simulink model "PID_SingleTank"  (R2016b)
settings: Solver=ode5  StartTime=0.0  StopTime=600  FixedStep=0.1  MaxStep=0.1  RelTol=1e-3
PreLoadFcn:
  | FuzzyK=readfis('FuzzySugenoPID_SingleTank.fis');
StartFcn:
  | FuzzyK=readfis('FuzzySugenoPID_SingleTank.fis');
Description:
  | The model describes dynamic properties of tank level system. The differential equation is:
  |                                            d/dt{Ah(t))=ku(t)-a*sqrt(2*g*h(t))
settings Model: ExtModeTrigMode=oneshot  ExtModeArmWhenConnect=off  Creator=Huynh Thai Hoang  LastModifiedBy=HTH
settings SolverCC: InitialStep=0.1
settings DataIOCC: SaveFormat=Array  SignalLoggingSaveFormat=ModelDataLogs  SaveOutput=off  SaveTime=off  SignalLoggingName=sigsOut
settings OptimizationCC: BooleanDataType=off  ExpressionDepthLimit=2147483647  LifeSpan=inf
settings DebuggingCC: SaveWithParameterizedLinksMsg=none  UnderspecifiedInitializationDetection=Classic  MergeDetectMultiDrivingBlocksExec=none  SignalResolutionControl=TryResolveAllWithWarning  MultiTaskDSMMsg=warning  MultiTaskCondExecSysMsg=none  FcnCallInpInsideContextMsg=warning  StateNameClashWarn=warning  SFUnexpectedBacktrackingDiag=warning  SFNoUnconditionalDefaultTransitionDiag=warning  SFExecutionAtInitializationDiag=none
settings HardwareCC: ProdBitPerPointer=32  ProdBitPerSizeT=32  ProdBitPerPtrDiffT=32  ProdLargestAtomicFloat=None  ProdIntDivRoundTo=Undefined  ProdEndianess=Unspecified  ProdWordSize=32  ProdHWDeviceType=32-bit Generic  TargetUnknown=on
settings ModelReferenceCC: PropagateSignalLabelsOutOfModel=off
settings GRTTargetCC: TargetLangStandard=C89/C90 (ANSI)  GeneratePreprocessorConditionals=Disable all  CombineOutputUpdateFcns=off  GRTInterface=on
settings ConfigComp: CovMetricSettings=dw  CovHtmlReporting=on  CovSaveCumulativeToWorkspaceVar=on  CovSaveSingleToWorkspaceVar=on  CovExternalEMLEnable=off

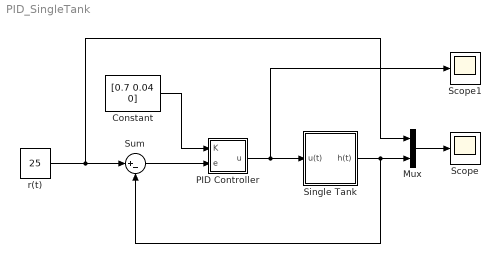
== system PID_SingleTank ==
  Constant : Constant  Value=[0.7 0.04 0]
  Mux : Mux  Inputs=2
  PID Controller : Subsystem  AncestorBlock=simulink_extras/Additional Linear/PID Controller  mask(PID Controller){}
      mask help:
      | Enter expressions for proportional, integral, and derivative terms.
      | P+I/s+Ds
      mask Help: This block implements a PID controller where parameters are entered for the Proportional, Integral and Derivative terms. Unmask this block to see how it works. The derivative term is implemented using a true derivative block.
  Scope : Scope
  Scope1 : Scope
  Single Tank : Subsystem  mask{A_min=50, A_max=200, a_out=1, h_max=50, Q_max=300, U_max=12, C=0.6}
      mask prompts: A_min "Minimum cross area (cm2)"; A_max "Maximum cross area (cm2)"; a_out "Outlet area (cm2)"; h_max "Tank height (cm)"; Q_max "Maximum pump flow (cm3/sec)"; U_max "Maximum control voltage (V)"; C "Discharge constant"
      mask init:
      | g=981;
      | k=Q_max/U_max;
      mask Display:
      | plot([0.1 0.3 0.9],[0.9 0.1 0.1]);
      | plot([0.9 0.7 0.9],[0.9 0.2 0.2]);
  Sum : Sum  Inputs=|+-  SaturateOnIntegerOverflow=on
  r(t) : Constant  Value=25
  wires:
  r(t)/1 -> Sum/1, Mux/1
  Sum/1 -> PID Controller/2(e)
  PID Controller/1(u) -> Single Tank/1(u(t)), Scope1/1
  Single Tank/1(h(t)) -> Sum/2, Mux/2
  Constant/1 -> PID Controller/1(K)
  Mux/1 -> Scope/1

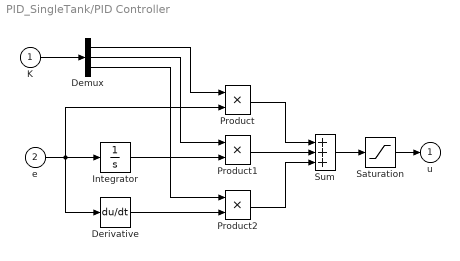
== system PID_SingleTank/PID Controller ==
  K : Inport
  e : Inport  Port=2
  Demux : Demux  Outputs=3
  Derivative : Derivative
  Integrator : Integrator
  Product : Product  SaturateOnIntegerOverflow=on  OutDataTypeStr=Inherit: Same as first input
  Product1 : Product  SaturateOnIntegerOverflow=on  OutDataTypeStr=Inherit: Same as first input
  Product2 : Product  SaturateOnIntegerOverflow=on  OutDataTypeStr=Inherit: Same as first input
  Saturation : Saturate  UpperLimit=12  LowerLimit=0
  Sum : Sum  Inputs=+++  SaturateOnIntegerOverflow=on  InputSameDT=on  OutDataTypeStr=Inherit: Same as first input
  u : Outport  InitialOutput=0
  wires:
  Product/1 -> Sum/1
  e/1 -> Product/2, Integrator/1, Derivative/1
  Sum/1 -> Saturation/1
  K/1 -> Demux/1
  Demux/1 -> Product/1
  Product1/1 -> Sum/2
  Integrator/1 -> Product1/2
  Demux/2 -> Product1/1
  Derivative/1 -> Product2/2
  Product2/1 -> Sum/3
  Demux/3 -> Product2/1
  Saturation/1 -> u/1

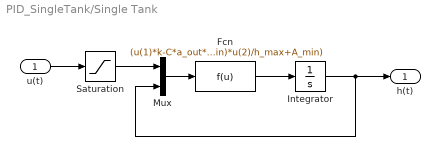
== system PID_SingleTank/Single Tank ==
  u(t) : Inport
  Fcn : Fcn  Expr=(u(1)*k-C*a_out*sqrt(2*g*u(2)))/((A_max-A_min)*u(2)/h_max+A_min)
  Integrator : Integrator  LimitOutput=on  UpperSaturationLimit=h_max  LowerSaturationLimit=0
  Mux : Mux  Inputs=2
  Saturation : Saturate  UpperLimit=12  LowerLimit=0
  h(t) : Outport
  wires:
  u(t)/1 -> Saturation/1
  Mux/1 -> Fcn/1
  Fcn/1 -> Integrator/1
  Integrator/1 -> h(t)/1, Mux/2
  Saturation/1 -> Mux/1
